simulink model "PV_Finall"  (Simulink 9.0)
settings: Solver=VariableStepAuto  StartTime=0.0  StopTime=10.0  RelTol=1e-3
libraries: simulink x3
settings Model: Creator=User  LastModifiedBy=User
settings DataIOCC: SaveFormat=Dataset
settings OptimizationCC: LifeSpan=auto
settings DebuggingCC: UnderspecifiedInitializationDetection=Simplified  MergeDetectMultiDrivingBlocksExec=error  SFUnexpectedBacktrackingDiag=error  SFNoUnconditionalDefaultTransitionDiag=error  SFExecutionAtInitializationDiag=warning
settings HardwareCC: ProdBitPerPointer=64  ProdBitPerSizeT=64  ProdBitPerPtrDiffT=64  ProdLargestAtomicFloat=Float  ProdIntDivRoundTo=Zero  ProdEndianess=LittleEndian  ProdWordSize=64  ProdHWDeviceType=Intel->x86-64 (Windows64)
settings ModelReferenceCC: PropagateSignalLabelsOutOfModel=on
settings CodeAppCC: StateflowObjectComments=off
settings GRTTargetCC: TargetLangStandard=C99 (ISO)
settings ConfigComp: CovMetricSettings=dwe  CovHtmlReporting=off  CovSaveCumulativeToWorkspaceVar=off  CovSaveSingleToWorkspaceVar=off  CovExternalEMLEnable=on

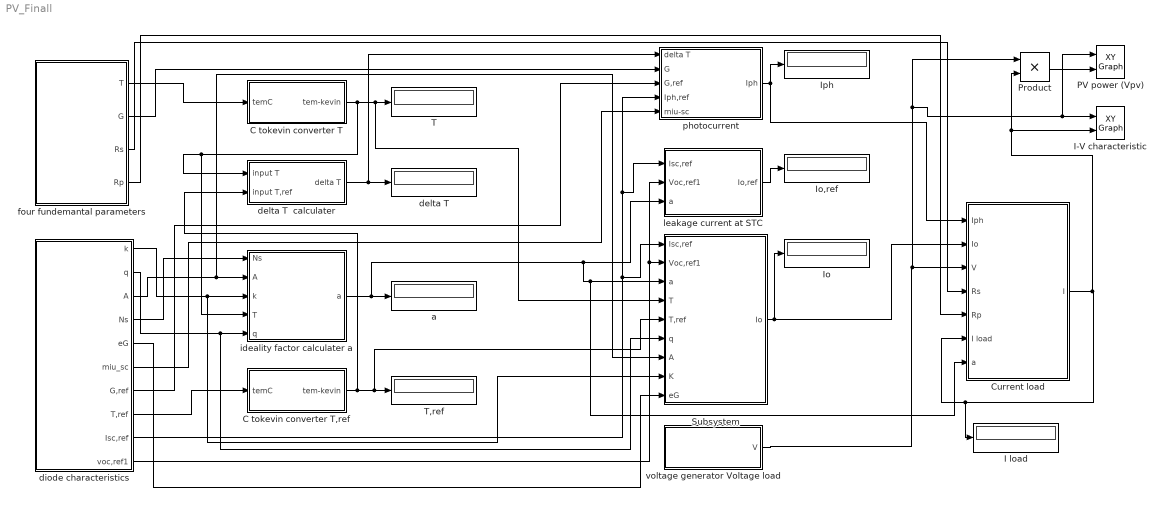
== system PV_Finall ==
  "C tokevin converter T " : Subsystem
  C tokevin converter T,ref : Subsystem
  Current load : Subsystem
  I load : Display
  I-V characteristic : simulink/Sinks/XY Graph  xmin=0  xmax=25  ymin=0  ymax=4  st=-1
  Io : Display
  Io,ref : Display
  Iph : Display
  PV power (Vpv) : simulink/Sinks/XY Graph  xmin=0  xmax=25  ymin=0  ymax=70  st=-1
  Product : Product  RndMeth=Zero
  Subsystem : Subsystem
  T : Display
  T,ref : Display
  a : Display
  delta T : Display
  delta T  calculater : Subsystem
  "diode characteristics " : Subsystem
  four fundemantal parameters : Subsystem
  ideality factor calculater a : Subsystem
  leakage current at STC : Subsystem
  photocurrent : Subsystem
  voltage generator Voltage load : Subsystem
  wires:
  delta T  calculater/1(delta T) -> photocurrent/1(delta T), delta T/1
  "diode characteristics "/4(Ns) -> ideality factor calculater a/1(Ns)
  "diode characteristics "/3(A) -> Subsystem/7(A), ideality factor calculater a/2(A)
  "diode characteristics "/1(k) -> Subsystem/8("K "), ideality factor calculater a/3(k)
  "diode characteristics "/2(q) -> Subsystem/6(q), ideality factor calculater a/5(q)
  four fundemantal parameters/1(T) -> "C tokevin converter T "/1(temC)
  "C tokevin converter T "/1(tem-kevin) -> Subsystem/4(T), T/1, ideality factor calculater a/4(T), delta T  calculater/1(input T)
  "diode characteristics "/8(T,ref) -> C tokevin converter T,ref/1(temC)
  C tokevin converter T,ref/1(tem-kevin) -> Subsystem/5(T,ref), T,ref/1, delta T  calculater/2(input T,ref)
  ideality factor calculater a/1(a) -> Current load/7(a), Subsystem/3(a), leakage current at STC/3(a), a/1
  four fundemantal parameters/2(G) -> photocurrent/2(G)
  "diode characteristics "/7(G,ref) -> photocurrent/3(G,ref)
  "diode characteristics "/6(miu_sc) -> photocurrent/5(miu-sc)
  "diode characteristics "/9(Isc,ref) -> Subsystem/1(Isc,ref), leakage current at STC/1(Isc,ref), photocurrent/4(Iph,ref)
  photocurrent/1(Iph) -> Current load/1("Iph "), Iph/1
  "diode characteristics "/10(voc,ref1) -> Subsystem/2(Voc,ref1), leakage current at STC/2(Voc,ref1)
  leakage current at STC/1(Io,ref) -> Io,ref/1
  Subsystem/1(Io) -> Io/1, Current load/2(Io)
  "diode characteristics "/5(eG) -> Subsystem/9(eG)
  voltage generator Voltage load/1(V) -> PV power (Vpv)/1, I-V characteristic/1, Product/1, Current load/3(V)
  four fundemantal parameters/4(Rp) -> Current load/5(Rp)
  four fundemantal parameters/3(Rs) -> Current load/4(Rs)
  Product/1 -> PV power (Vpv)/2
  Current load/1(I) -> Product/2, I-V characteristic/2, I load/1, Current load/6("I load ")

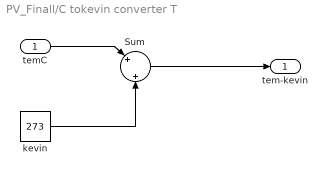
== system PV_Finall/C tokevin converter T  ==
  temC : Inport
  Sum : Sum  Inputs=|+||+
  kevin : Constant  Value=273
  tem-kevin : Outport
  wires:
  temC/1 -> Sum/1
  Sum/1 -> tem-kevin/1
  kevin/1 -> Sum/2

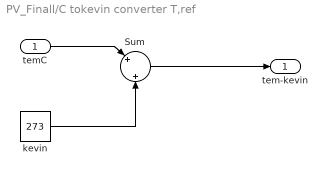
== system PV_Finall/C tokevin converter T,ref ==
  temC : Inport
  Sum : Sum  Inputs=|+||+
  kevin : Constant  Value=273
  tem-kevin : Outport
  wires:
  temC/1 -> Sum/1
  Sum/1 -> tem-kevin/1
  kevin/1 -> Sum/2

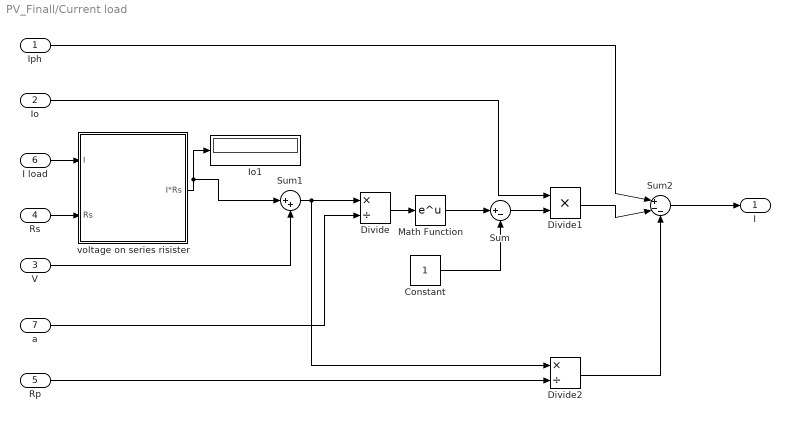
== system PV_Finall/Current load ==
  "Iph " : Inport
  Io : Inport  Port=2
  V : Inport  Port=3
  Rs : Inport  Port=4
  Rp : Inport  Port=5
  "I load " : Inport  Port=6
  a : Inport  Port=7
  Constant : Constant
  Divide : Product  Inputs=*/
  Divide1 : Product
  Divide2 : Product  Inputs=*/
  Io1 : Display
  Math Function : Math  SaturateOnIntegerOverflow=on
  Sum : Sum  Inputs=|+-
  Sum1 : Sum  Inputs=|++
  Sum2 : Sum  Inputs=|+--
  voltage on series risister : Subsystem
  I : Outport
  wires:
  "I load "/1 -> voltage on series risister/1(I)
  Rs/1 -> voltage on series risister/2(Rs)
  voltage on series risister/1(I*Rs) -> Sum1/1, Io1/1
  V/1 -> Sum1/2
  Sum1/1 -> Divide2/1, Divide/1
  a/1 -> Divide/2
  Divide/1 -> Math Function/1
  Math Function/1 -> Sum/1
  Constant/1 -> Sum/2
  Sum/1 -> Divide1/2
  Io/1 -> Divide1/1
  Rp/1 -> Divide2/2
  "Iph "/1 -> Sum2/1
  Divide1/1 -> Sum2/2
  Divide2/1 -> Sum2/3
  Sum2/1 -> I/1

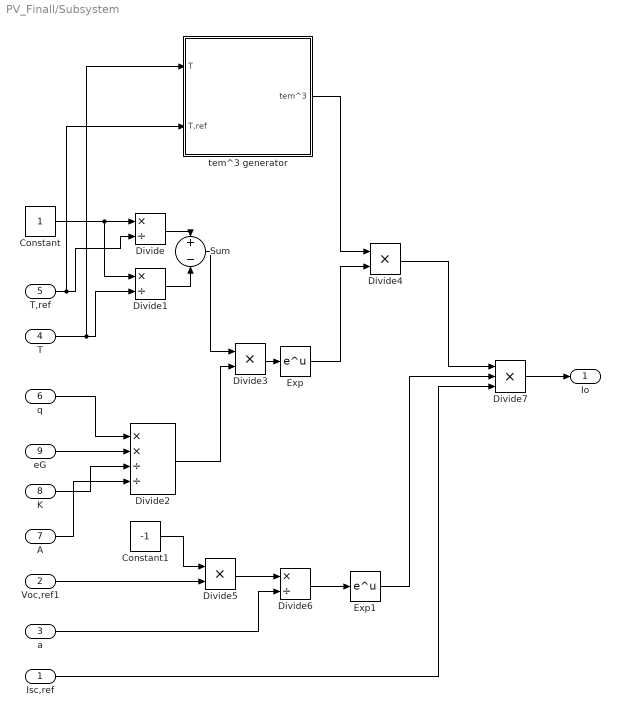
== system PV_Finall/Subsystem ==
  Isc,ref : Inport
  Voc,ref1 : Inport  Port=2
  a : Inport  Port=3
  T : Inport  Port=4
  T,ref : Inport  Port=5
  q : Inport  Port=6
  A : Inport  Port=7
  "K " : Inport  Port=8
  eG : Inport  Port=9
  Constant : Constant
  Constant1 : Constant  Value=-1
  Divide : Product  Inputs=*/
  Divide1 : Product  Inputs=*/
  Divide2 : Product  Inputs=**//
  Divide3 : Product  Inputs=**
  Divide4 : Product  Inputs=**
  Divide5 : Product  Inputs=**
  Divide6 : Product  Inputs=*/
  Divide7 : Product  Inputs=3
  Exp : Math  SaturateOnIntegerOverflow=on
  Exp1 : Math  SaturateOnIntegerOverflow=on
  Sum : Sum  Inputs=+|-
  tem^3 generator : Subsystem
  Io : Outport
  wires:
  T/1 -> tem^3 generator/1(T), Divide1/2
  T,ref/1 -> tem^3 generator/2(T,ref), Divide/2
  Constant/1 -> Divide1/1, Divide/1
  Divide/1 -> Sum/1
  Divide1/1 -> Sum/2
  q/1 -> Divide2/1
  eG/1 -> Divide2/2
  "K "/1 -> Divide2/3
  A/1 -> Divide2/4
  Sum/1 -> Divide3/1
  Divide2/1 -> Divide3/2
  Divide3/1 -> Exp/1
  tem^3 generator/1(tem^3) -> Divide4/1
  Exp/1 -> Divide4/2
  Voc,ref1/1 -> Divide5/2
  Constant1/1 -> Divide5/1
  Divide5/1 -> Divide6/1
  a/1 -> Divide6/2
  Divide6/1 -> Exp1/1
  Isc,ref/1 -> Divide7/3
  Exp1/1 -> Divide7/2
  Divide4/1 -> Divide7/1
  Divide7/1 -> Io/1

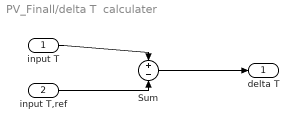
== system PV_Finall/delta T  calculater ==
  input T : Inport
  input T,ref : Inport  Port=2
  Sum : Sum  Inputs=+|-
  delta T : Outport
  wires:
  input T/1 -> Sum/1
  input T,ref/1 -> Sum/2
  Sum/1 -> delta T/1

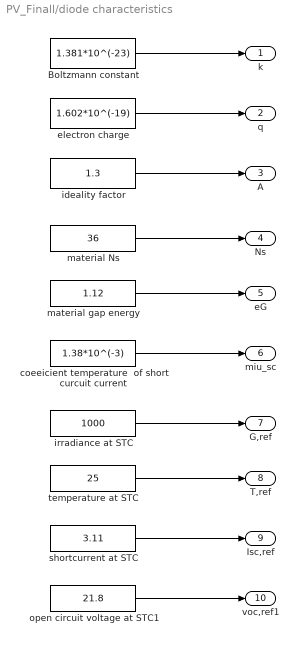
== system PV_Finall/diode characteristics  ==
  Boltzmann constant : Constant  Value=1.381*10^(-23)
  coeeicient temperature  of short curcuit current : Constant  Value=1.38*10^(-3)
  electron charge : Constant  Value=1.602*10^(-19)
  ideality factor : Constant  Value=1.3
  irradiance at STC : Constant  Value=1000
  material Ns : Constant  Value=36
  material gap energy : Constant  Value=1.12
  open circuit voltage at STC1 : Constant  Value=21.8
  shortcurrent at STC : Constant  Value=3.11
  temperature at STC : Constant  Value=25
  k : Outport
  q : Outport  Port=2
  A : Outport  Port=3
  Ns : Outport  Port=4
  eG : Outport  Port=5
  miu_sc : Outport  Port=6
  G,ref : Outport  Port=7
  T,ref : Outport  Port=8
  Isc,ref : Outport  Port=9
  voc,ref1 : Outport  Port=10
  wires:
  Boltzmann constant/1 -> k/1
  electron charge/1 -> q/1
  ideality factor/1 -> A/1
  material Ns/1 -> Ns/1
  material gap energy/1 -> eG/1
  coeeicient temperature  of short curcuit current/1 -> miu_sc/1
  irradiance at STC/1 -> G,ref/1
  temperature at STC/1 -> T,ref/1
  shortcurrent at STC/1 -> Isc,ref/1
  open circuit voltage at STC1/1 -> voc,ref1/1

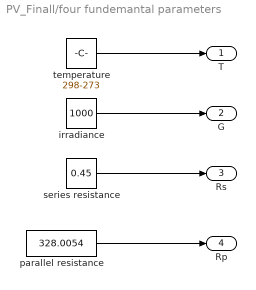
== system PV_Finall/four fundemantal parameters ==
  irradiance : Constant  Value=1000
  parallel resistance : Constant  Value=328.0054
  series resistance : Constant  Value=0.45
  temperature : Constant  Value=298-273
  T : Outport
  G : Outport  Port=2
  Rs : Outport  Port=3
  Rp : Outport  Port=4
  wires:
  temperature/1 -> T/1
  irradiance/1 -> G/1
  series resistance/1 -> Rs/1
  parallel resistance/1 -> Rp/1

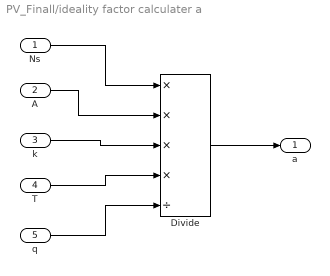
== system PV_Finall/ideality factor calculater a ==
  Ns : Inport
  A : Inport  Port=2
  k : Inport  Port=3
  T : Inport  Port=4
  q : Inport  Port=5
  Divide : Product  Inputs=****/
  a : Outport
  wires:
  Ns/1 -> Divide/1
  A/1 -> Divide/2
  k/1 -> Divide/3
  T/1 -> Divide/4
  q/1 -> Divide/5
  Divide/1 -> a/1

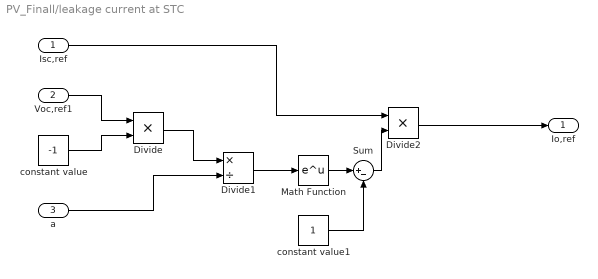
== system PV_Finall/leakage current at STC ==
  Isc,ref : Inport
  Voc,ref1 : Inport  Port=2
  a : Inport  Port=3
  Divide : Product
  Divide1 : Product  Inputs=*/
  Divide2 : Product
  Math Function : Math  SaturateOnIntegerOverflow=on
  Sum : Sum  Inputs=|+-
  constant value : Constant  Value=-1
  constant value1 : Constant
  Io,ref : Outport
  wires:
  Voc,ref1/1 -> Divide/1
  constant value/1 -> Divide/2
  Divide/1 -> Divide1/1
  a/1 -> Divide1/2
  Divide1/1 -> Math Function/1
  Isc,ref/1 -> Divide2/1
  Divide2/1 -> Io,ref/1
  Math Function/1 -> Sum/1
  Sum/1 -> Divide2/2
  constant value1/1 -> Sum/2

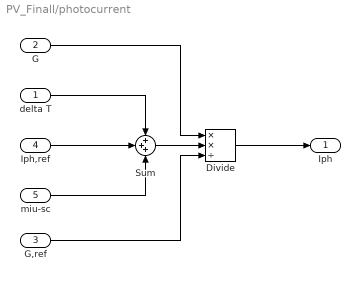
== system PV_Finall/photocurrent ==
  delta T : Inport
  G : Inport  Port=2
  G,ref : Inport  Port=3
  Iph,ref : Inport  Port=4
  miu-sc : Inport  Port=5
  Divide : Product  Inputs=**/
  Sum : Sum  Inputs=3
  Iph : Outport
  wires:
  delta T/1 -> Sum/1
  Iph,ref/1 -> Sum/2
  miu-sc/1 -> Sum/3
  G/1 -> Divide/1
  G,ref/1 -> Divide/3
  Sum/1 -> Divide/2
  Divide/1 -> Iph/1

== system PV_Finall/voltage generator Voltage load ==
  "V      " : simulink/Sources/Repeating Sequence  rep_seq_t=[0 1 2]  rep_seq_y="[0  21.5 0]"
  V : Outport
  wires:
  "V      "/1 -> V/1

== system PV_Finall/Current load/voltage on series risister ==
  I : Inport
  Rs : Inport  Port=2
  Divide : Product
  I*Rs : Outport
  wires:
  I/1 -> Divide/1
  Rs/1 -> Divide/2
  Divide/1 -> I*Rs/1

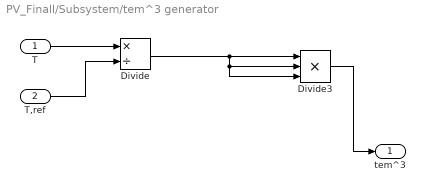
== system PV_Finall/Subsystem/tem^3 generator ==
  T : Inport
  T,ref : Inport  Port=2
  Divide : Product  Inputs=*/
  Divide3 : Product  Inputs=3
  tem^3 : Outport
  wires:
  Divide/1 -> Divide3/3, Divide3/2, Divide3/1
  Divide3/1 -> tem^3/1
  T/1 -> Divide/1
  T,ref/1 -> Divide/2
